simulink model "p1"  (R2020b)
settings: Solver=VariableStepAuto  StartTime=0.0  StopTime=10.0  RelTol=1e-3
model workspace (MAT data in the model file):
  M1 = 100
  M2 = 50
  b = 50
  k1 = 50
  k12 = 25
settings Model: Creator=mluser  LastModifiedBy=mluser

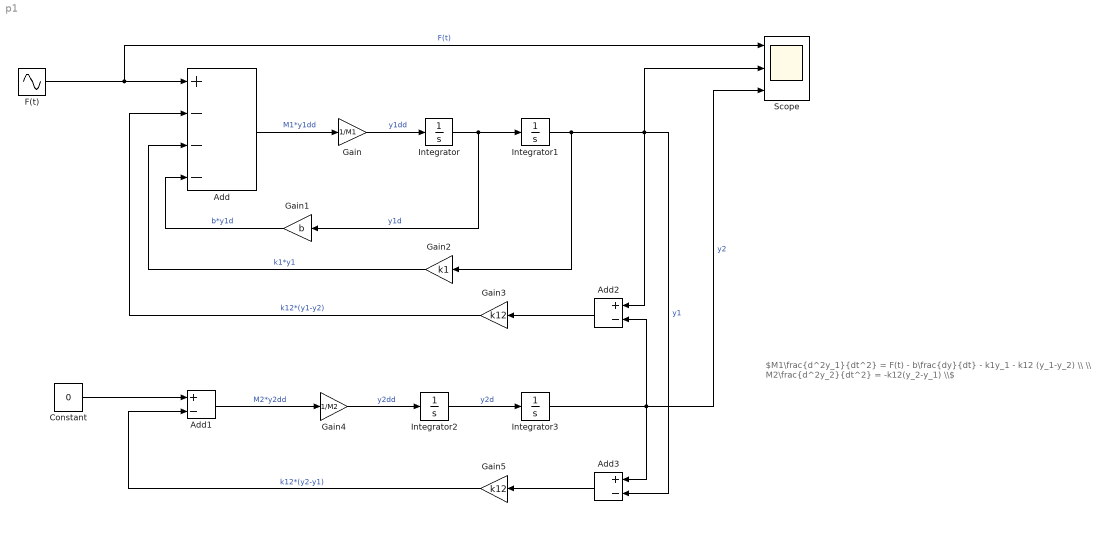
== system p1 ==
  note: $M1\frac{d^2y_1}{dt^2} = F(t) - b\frac{dy}{dt} - k1y_1 - k12 (y_1-y_2) \\ \\ M2\frac{d^2y_2}{dt^2} = -k12(y_2-y_1) \\$
  Add : Sum  Inputs=+---
  Add1 : Sum  Inputs=+-
  Add2 : Sum  Inputs=+-
  Add3 : Sum  Inputs=+-
  Constant : Constant  Value=0
  F(t) : Sin  Amplitude=2  Frequency=10/(2*pi)  SampleTime=0
  Gain : Gain  Gain=1/M1
  Gain1 : Gain  Gain=b
  Gain2 : Gain  Gain=k1
  Gain3 : Gain  Gain=k12
  Gain4 : Gain  Gain=1/M2
  Gain5 : Gain  Gain=k12
  Integrator{,1..3} (4 alike) : Integrator
  Scope : Scope  NumInputPorts=3
  wires:
  F(t)/1 -> Scope/1, Add/1  "F(t)"
  Integrator1/1 -> Add2/1, Add3/2, Scope/2, Gain2/1  "y1"
  Add/1 -> Gain/1  "M1*y1dd"
  Add2/1 -> Gain3/1
  Integrator2/1 -> Integrator3/1  "y2d"
  Add3/1 -> Gain5/1
  Gain1/1 -> Add/4  "b*y1d"
  Gain3/1 -> Add/2  "k12*(y1-y2)"
  Gain2/1 -> Add/3  "k1*y1"
  Add1/1 -> Gain4/1  "M2*y2dd"
  Integrator3/1 -> Scope/3, Add3/1, Add2/2  "y2"
  Integrator/1 -> Gain1/1, Integrator1/1  "y1d"
  Gain5/1 -> Add1/2  "k12*(y2-y1)"
  Constant/1 -> Add1/1
  Gain4/1 -> Integrator2/1  "y2dd"
  Gain/1 -> Integrator/1  "y1dd"
